simulink model "controller_template_ObsAvoid"  (Simulink 7.8)
settings: Solver=FixedStepDiscrete  SolverMode=SingleTasking  StartTime=0.0  StopTime=inf  FixedStep=Ts  RelTol=1e-3
PreLoadFcn:
  | load_waypoints
  | main;
StopFcn:
  | y_ref_wall = RecordYZ.signals(1).values(:,2);
  | y_wall = RecordYZ.signals(1).values(:,1);
  | 
  | z_ref_wall = RecordYZ.signals(2).values(:,2);
  | z_wall = RecordYZ.signals(2).values(:,1);
  | 
  | close all;
  | figure;
  | plot(y_ref_wall,z_ref_wall,'b','LineWidth',2); hold on;
  | plot(y_wall,z_wall,'r','LineWidth',2); grid on;
  | plot(traj_FG.X_ref_y_real(1,:),-traj_FG.X_ref_z_real(1,:),'o-g');
  | axis equal;
values from neighbouring files (symbols this model uses):
  Fi_Yaw = [-1.14619813144 0 0]    [kostas_malakies.mat]    (also in kostas_malakies2.mat; matlab.mat = -0.284754025426)
  Fi_Zdir = [0 -1.80359099426e-16 0 1.4149586889 0 0 2.30859647265e-14 -5.77149118162e-15 0 0 0 0 ... (54 elements, 27x2)]    [kostas_malakies.mat]    (also in kostas_malakies2.mat = [4.30976351396 0 4.73307471514 3.80948040666 0 0 0 0.5468933; matlab.mat = [0 -9.51943523339e-14 0 1.99761158231 0 1.18992940417e-14 0 )
  g = 9.8065    [kostas_malakies.mat]    (also in kostas_malakies2.mat; load_PMModel.m = 9.81; main.m; main_last.m)
  Gi_Yaw = [4.4408920985e-16 -3.14159265359 3.14159265359]    [kostas_malakies.mat]    (also in kostas_malakies2.mat = [-4.4408920985e-16 -3.14159265359 3.14159265359]; matlab.mat = 4.4408920985e-16)
  Gi_Zdir = [-1 -1 -1 2.22044604925e-16 -1 -1 -1 -1 1 -1 -1 -1 ... (27 elements, 27x1)]    [kostas_malakies.mat]    (also in kostas_malakies2.mat = [0.174387892495 -1 0.368373831608 3.33066907388e-16 -1 -1 -1; matlab.mat = [-2 -2 -2 1.11022302463e-15 -2 -2 -2 2 -2 -2 -2 2 ... (21 el)
  Hn_Yaw = [1 -1 -1 1 1 -1]    [kostas_malakies.mat]    (also in kostas_malakies2.mat; matlab.mat = [1 -1])
  Hn_Zdir = [-0.560552458797 -0.996815278536 -0.988320507921 0.666673243042 -1 0 -0.421994354267 -0.987440631917 -0.973284290019 -0.956170964903 -0.936236606521 0.560552458797 ... (224 elements, 112x2)]    [kostas_malakies.mat]    (also in kostas_malakies2.mat = [-0.781813705838 -0.712499731132 0.751798766698 0 -0.7286973; matlab.mat = [1 -1 -0.996815278536 -0.990718937584 -0.276007160242 0.3840)
  kalm_mpc_yaw =     [kostas_malakies.mat]    (also in kostas_malakies2.mat)
  Kn_Yaw = [2.74088097634 2.74088097634 -2.74088097634 3.14159265359 -2.74088097634 3.14159265359]    [kostas_malakies.mat]    (also in kostas_malakies2.mat; matlab.mat = [0.0873 0.0873])
  Kn_Zdir = [0.727672356179 1.00172267683 1.00656919451 -0.471160923828 1 1 1.18526984431 1.00688561667 1.01272393898 1.01603878926 1.01572683497 -0.727672356179 ... (112 elements, 112x1)]    [kostas_malakies.mat]    (also in kostas_malakies2.mat = [0.21304012328 0.326509029469 -0.262060822346 1 0.301409884 ; matlab.mat = [1 1 1.00663007512 1.02122194908 0.632590992205 -0.384463644)
  MAX_BIAS_YAW_RATE = 0.0872664625997    [kostas_malakies.mat]    (also in kostas_malakies2.mat; main.m; main_last.m)
  Nc_Yaw = [2 2 2]    [kostas_malakies.mat]    (also in kostas_malakies2.mat; matlab.mat = 2)
  Nc_Zdir = [6 7 3 6 3 4 4 3 6 5 3 4 ... (27 elements, 27x1)]    [kostas_malakies.mat]    (also in kostas_malakies2.mat = [4 4 3 12 5 4 3 3 4 3 3 4 ... (93 elements, 93x1)]; matlab.mat = [6 3 7 4 4 3 4 6 3 5 3 3 ... (21 elements, 21x1)])
  pitch_cmd2pitch_1stOrd = 1.42468924998    [kostas_malakies.mat]    (also in kostas_malakies2.mat)
  roll_cmd2roll_1stOrd = 1.38101661575    [kostas_malakies.mat]    (also in kostas_malakies2.mat)
  thrust_cmd2thrust_0thOrd = 0.876575459522    [kostas_malakies.mat]    (also in kostas_malakies2.mat)
  THRUST_CMD_GAIN = -0.0835    [kostas_malakies.mat]    (also in kostas_malakies2.mat; load_PMModel.m)
  traj_FG =     [kostas.mat]    (also in kostas_malakies.mat; kostas_malakies2.mat; main.m = ReferenceCreator(maxdisty,maxdistz,scale_y,scale_z); main_last.m = ReferenceCreator(maxdisty,maxdistz,scale_y,scale_z))
  Ts = 0.02    [kostas_malakies.mat]    (also in kostas_malakies2.mat; main.m; main_last.m; matlab.mat = 0.08)
  yaw_cmd2yaw_1stOrd = 2.01792090263    [kostas_malakies.mat]    (also in kostas_malakies2.mat)
  z = [-0.93079906702 -0.933865725994 -0.937557637691 -0.939011216164 -0.94143640995 -0.944628417492 -0.947235524654 -0.949601888657 -0.952827751637 -0.9567258358 -0.958320975304 -0.960991024971 ... (7988 elements, 7988x1)]    [kostas_malakies2.mat]    (also in plotDataTest.m = simout_data.signals.values(:,11))
undefined symbols (not defined in the file or in its folder): XYctrl
libraries: simulink x44, Hquad_control_LIB_MPC x13
(part 2 of 2)

== system controller_template_ObsAvoid/FreeFlight Pos Ctrl/MAIN CONTROL LOOP1/z controller MPC FG ==
  reset : Inport  PortDimensions=1
  X_ref_z : Inport  Port=2
  "z_states_est  " : Inport  Port=3
  Add : Sum  Inputs=+-
  Demux : Demux  Outputs=3
  Display : Display
  Display1 : Display
  Explicit Ctrl1 : Subsystem
  Mean : Subsystem
  Mux : Mux  Inputs=3
  Saturation : Saturate  UpperLimit=1  LowerLimit=-1
  Saturation1 : Saturate  UpperLimit=1  LowerLimit=-1
  Saturation2 : Saturate  UpperLimit=1  LowerLimit=-1
  Slider Gain : simulink/Math Operations/Slider Gain  low=0  gain=1.1  high=2
  Subsystem : Subsystem
  Wall Deviation : Subsystem
  thrust_cmd : Outport  PortDimensions=1
  wires:
  "z_states_est  "/1 -> Demux/1
  Demux/2 -> Saturation/1
  Demux/1 -> Add/1
  X_ref_z/1 -> Add/2
  Add/1 -> Saturation1/1
  Mux/1 -> Explicit Ctrl1/1(States)
  Saturation/1 -> Mux/2
  Saturation1/1 -> Display/1, Mux/1, Subsystem/3(dz)
  Mean/1(u_mean) -> thrust_cmd/1, Display1/1
  Saturation2/1 -> Mean/1(u)
  Demux/3 -> Wall Deviation/1(posx)
  Wall Deviation/1(deltax) -> Mux/3, Subsystem/2(dx)
  Explicit Ctrl1/1(Input) -> Subsystem/1(u_thrust)
  Subsystem/1(u_thrust_out) -> Slider Gain/1
  Slider Gain/1 -> Saturation2/1

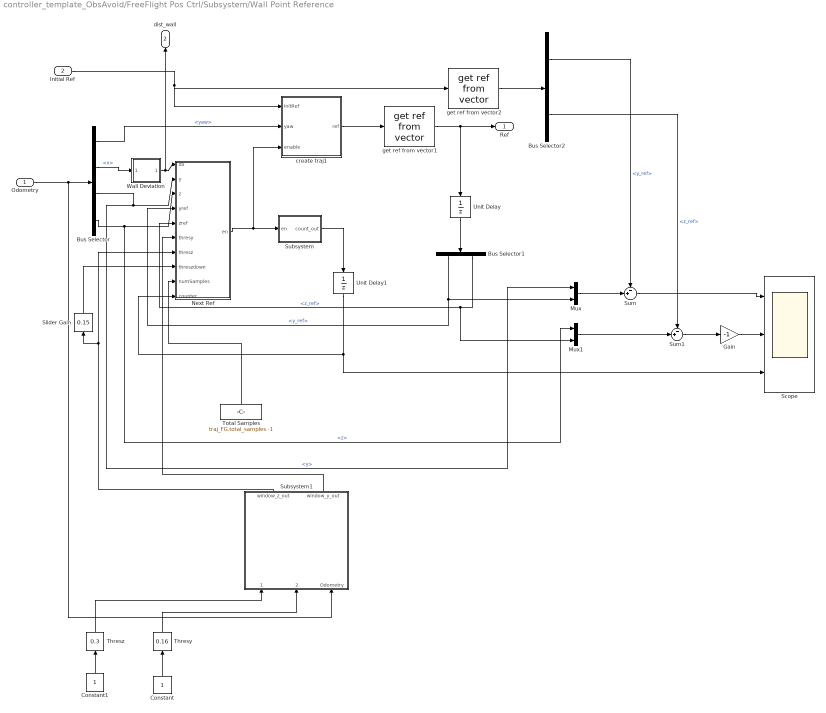
== system controller_template_ObsAvoid/FreeFlight Pos Ctrl/Subsystem/Wall Point Reference ==
  Odometry : Inport
  Initial Ref : Inport  Port=2
  Bus Selector : BusSelector  OutputSignals=rpy.yaw,pos.x,pos.y,pos.z
  Bus Selector1 : BusSelector  OutputSignals=pose_ref.y_ref,pose_ref.z_ref
  Bus Selector2 : BusSelector  OutputSignals=pose_ref.y_ref,pose_ref.z_ref
  Constant : Constant
  Constant1 : Constant
  Gain : Gain  Gain=-1
  Mux : Mux  Inputs=2
  Mux1 : Mux  Inputs=2
  Next Ref : MATLAB Function  TreatAsAtomicUnit=on
  Scope : Scope  NumInputPorts=3
      settings: YMin=0.575~-0.125~58  YMax=1.125~0.275~64  SaveName=RecordYZ
  Slider Gain : simulink/Math Operations/Slider Gain  low=0  gain=0.15  high=2
  Subsystem : Subsystem
  Subsystem1 : Subsystem
  Sum : Sum  Inputs=-+|
  Sum1 : Sum  Inputs=-+|
  Thresy : simulink/Math Operations/Slider Gain  low=0  gain=0.16  high=1
  Thresz : simulink/Math Operations/Slider Gain  low=0  gain=0.3  high=2
  Total Samples : Constant  Value=traj_FG.total_samples -1
  Unit Delay : UnitDelay  SampleTime=-1
  Unit Delay1 : UnitDelay  SampleTime=-1
  Wall Deviation : Subsystem
  create traj1 : Subsystem
  get ref from vector1 : Hquad_control_LIB_MPC/pos controller/get ref from vector
  get ref from vector2 : Hquad_control_LIB_MPC/pos controller/get ref from vector
  Ref : Outport
  dist_wall : Outport  Port=2
  wires:
  get ref from vector1/1 -> Ref/1, Unit Delay/1
  create traj1/1(ref) -> get ref from vector1/1
  Initial Ref/1 -> create traj1/1(InitRef), get ref from vector2/1
  Odometry/1 -> Bus Selector/1, Subsystem1/3(Odometry)
  Bus Selector/1 -> create traj1/2(yaw)  "<yaw>"
  Bus Selector/3 -> Next Ref/2(y), Mux/1  "<y>"
  Bus Selector/4 -> Next Ref/3(z), Mux1/1  "<z>"
  Unit Delay/1 -> Bus Selector1/1
  Bus Selector1/1 -> Next Ref/4(yref), Mux/2  "<y_ref>"
  Bus Selector1/2 -> Next Ref/5(zref), Mux1/2  "<z_ref>"
  Constant/1 -> Thresy/1
  Thresy/1 -> Subsystem1/2(nominal_window_y)
  Next Ref/1(en) -> create traj1/3(enable), Subsystem/1(en)
  Wall Deviation/1(deltax) -> Next Ref/1(dx), dist_wall/1
  Bus Selector/2 -> Wall Deviation/1(posx)  "<x>"
  Total Samples/1 -> Next Ref/9(numSamples)
  Unit Delay1/1 -> Next Ref/10(counter), Scope/3
  Subsystem/1(count_out) -> Unit Delay1/1
  Constant1/1 -> Thresz/1
  Thresz/1 -> Subsystem1/1(nominal_window_z)
  Gain/1 -> Scope/2
  Mux/1 -> Sum/2
  Mux1/1 -> Sum1/2
  Sum1/1 -> Gain/1
  Sum/1 -> Scope/1
  get ref from vector2/1 -> Bus Selector2/1
  Bus Selector2/1 -> Sum/1  "<y_ref>"
  Bus Selector2/2 -> Sum1/1  "<z_ref>"
  Subsystem1/2(window_y_out) -> Next Ref/6(thresy)
  Subsystem1/1(window_z_out) -> Next Ref/7(thresz), Slider Gain/1
  Slider Gain/1 -> Next Ref/8(threszdown)

== system controller_template_ObsAvoid/FreeFlight Pos Ctrl/decoupling and rotation/decoupling  ==
  "roll_meas  " : Inport  PortDimensions=1
  "pitch_meas  " : Inport  Port=2  PortDimensions=1
  cmd : Inport  Port=3
  mass : Inport  Port=4
  posx : Inport  Port=5
  Bus Creator : BusCreator
  Bus Selector3 : BusSelector  OutputSignals=pitch_cmd,roll_cmd,thrust_cmd,yaw_rate_cmd
  Embedded MATLAB Function : MATLAB Function  TreatAsAtomicUnit=on
  Wall Deviation : Subsystem
  g : Constant  Value=g
  "cmd_comp  " : Outport
  wires:
  "roll_meas  "/1 -> Embedded MATLAB Function/2(roll_meas)
  "pitch_meas  "/1 -> Embedded MATLAB Function/1(pitch_meas)
  cmd/1 -> Bus Selector3/1
  Bus Selector3/4 -> Bus Creator/4  "<yaw_rate_cmd>"
  Bus Creator/1 -> "cmd_comp  "/1
  Embedded MATLAB Function/3(thrust_comp) -> Bus Creator/3  "thrust_cmd"
  Embedded MATLAB Function/2(roll_cmd_comp) -> Bus Creator/2  "roll_cmd"
  Embedded MATLAB Function/1(pitch_cmd_comp) -> Bus Creator/1  "pitch_cmd"
  Bus Selector3/1 -> Embedded MATLAB Function/3(pitch_cmd)  "<pitch_cmd>"
  Bus Selector3/2 -> Embedded MATLAB Function/4(roll_cmd)  "<roll_cmd>"
  Bus Selector3/3 -> Embedded MATLAB Function/5(thrust)  "<thrust_cmd>"
  mass/1 -> Embedded MATLAB Function/6(m)
  g/1 -> Embedded MATLAB Function/7(g)
  posx/1 -> Wall Deviation/1(posx)
  Wall Deviation/1(deltax) -> Embedded MATLAB Function/8(posx)

== system controller_template_ObsAvoid/FreeFlight Pos Ctrl/decoupling and rotation/rotate_to_quat_frame ==
  yaw_meas : Inport
  cmd_comp : Inport  Port=2
  bias : Inport  Port=3
  Bus Creator1 : BusCreator
  Bus Creator2 : BusCreator
  Bus Selector1 : BusSelector  OutputSignals=thrust_bias,yaw_rate_bias
  Bus Selector2 : BusSelector  OutputSignals=pitch_bias,roll_bias
  Bus Selector3 : BusSelector  OutputSignals=pitch_cmd,roll_cmd
  Bus Selector4 : BusSelector  OutputSignals=thrust_cmd,yaw_rate_cmd
  Embedded MATLAB Function : MATLAB Function  TreatAsAtomicUnit=on
  "cmd_rot  " : Outport
  bias_rot : Outport  Port=2
  wires:
  yaw_meas/1 -> Embedded MATLAB Function/1(yaw)
  bias/1 -> Bus Selector2/1, Bus Selector1/1
  Bus Creator1/1 -> bias_rot/1
  Bus Selector2/1 -> Embedded MATLAB Function/4(pitch_bias)  "<pitch_bias>"
  Bus Selector2/2 -> Embedded MATLAB Function/5(roll_bias)  "<roll_bias>"
  Embedded MATLAB Function/3(pitch_bias_rot) -> Bus Creator1/1  "pitch_bias"
  Embedded MATLAB Function/4(roll_bias_rot) -> Bus Creator1/2  "roll_bias"
  Bus Creator2/1 -> "cmd_rot  "/1
  Bus Selector3/2 -> Embedded MATLAB Function/3(roll_cmd)  "<roll_cmd>"
  Bus Selector3/1 -> Embedded MATLAB Function/2(pitch_cmd)  "<pitch_cmd>"
  cmd_comp/1 -> Bus Selector3/1, Bus Selector4/1
  Embedded MATLAB Function/1(pitch_rot) -> Bus Creator2/1  "pitch_cmd"
  Embedded MATLAB Function/2(roll_rot) -> Bus Creator2/2  "roll_cmd"
  Bus Selector4/1 -> Bus Creator2/3  "<thrust_cmd>"
  Bus Selector4/2 -> Bus Creator2/4  "<yaw_rate_cmd>"
  Bus Selector1/1 -> Bus Creator1/3  "<thrust_bias>"
  Bus Selector1/2 -> Bus Creator1/4  "<yaw_rate_bias>"

== system controller_template_ObsAvoid/pos controller/MAIN CONTROL LOOP1/demux ==
  odometry : Inport
  ref : Inport  Port=2
  reset : Inport  Port=3
  Bus Creator : BusCreator  Inputs=3
  Bus Creator1 : BusCreator  Inputs=3
  Bus Creator2 : BusCreator  Inputs=2
  Bus Creator3 : BusCreator  Inputs=2
  Bus Selector1 : BusSelector  OutputSignals=X_ref_x,X_ref_y,X_ref_z,X_ref_yaw
  Bus Selector2 : BusSelector  OutputSignals=pos.x,vel.x_dot,rpy.pitch,pos.y,vel.y_dot,rpy.roll,pos.z,vel.z_dot,rpy.yaw,ang_vel.ang_vel_z
  reset1 : Outport
  X_ref_x : Outport  Port=2
  x_states_meas : Outport  Port=3  PortDimensions=3
  reset2 : Outport  Port=4
  X_ref_y : Outport  Port=5
  y_states_meas : Outport  Port=6  PortDimensions=3
  reset3 : Outport  Port=7
  X_ref_z : Outport  Port=8
  z_states_meas : Outport  Port=9  PortDimensions=2
  reset4 : Outport  Port=10
  X_ref_yaw : Outport  Port=11
  yaw_states_meas : Outport  Port=12  PortDimensions=2
  wires:
  Bus Selector1/4 -> X_ref_yaw/1  "<X_ref_yaw>"
  Bus Selector1/3 -> X_ref_z/1  "<X_ref_z>"
  Bus Selector2/6 -> Bus Creator1/3  "<roll>"
  Bus Selector2/3 -> Bus Creator/3  "<pitch>"
  odometry/1 -> Bus Selector2/1
  Bus Creator/1 -> x_states_meas/1
  Bus Selector2/1 -> Bus Creator/1  "<x>"
  Bus Selector2/2 -> Bus Creator/2  "<x_dot>"
  Bus Selector2/4 -> Bus Creator1/1  "<y>"
  Bus Selector2/5 -> Bus Creator1/2  "<y_dot>"
  Bus Creator1/1 -> y_states_meas/1
  Bus Selector2/7 -> Bus Creator2/1  "<z>"
  Bus Selector2/8 -> Bus Creator2/2  "<z_dot>"
  Bus Selector2/9 -> Bus Creator3/1  "<yaw>"
  Bus Selector2/10 -> Bus Creator3/2  "<ang_vel_z>"
  Bus Creator2/1 -> z_states_meas/1
  Bus Creator3/1 -> yaw_states_meas/1
  ref/1 -> Bus Selector1/1
  Bus Selector1/1 -> X_ref_x/1  "<X_ref_x>"
  Bus Selector1/2 -> X_ref_y/1  "<X_ref_y>"
  reset/1 -> reset3/1, reset4/1, reset2/1, reset1/1

== system controller_template_ObsAvoid/pos controller/MAIN CONTROL LOOP1/yaw states estimator bias ==
  yaw_rate_cmd : Inport  PortDimensions=1
  yaw_states_meas : Inport  Port=2  PortDimensions=2
  yaw_rate_bias_in : Inport  Port=3  PortDimensions=1
  A : Constant  Value=kalm_mpc_yaw.A
  B : Constant  Value=kalm_mpc_yaw.B
  Bus Selector3 : BusSelector  OutputSignals=yaw,ang_vel_z
  C : Constant  Value=kalm_mpc_yaw.C
  D : Constant  Value=kalm_mpc_yaw.D
  Demux3 : Demux  Outputs=2
  Mux1 : Mux  Inputs=2
  Mux4 : Mux  Inputs=2
  Q : Constant  Value=kalm_mpc_yaw.Q
  R : Constant  Value=kalm_mpc_yaw.R
  Saturation : Saturate  UpperLimit=MAX_BIAS_YAW_RATE  LowerLimit=-MAX_BIAS_YAW_RATE
  Unit Delay External IC1 : simulink/Additional Math & Discrete/Additional Discrete/Unit Delay External IC  tsamp=-1
  Unit Delay1 : UnitDelay  X0=kalm_mpc_yaw.P  SampleTime=Ts
  discrete kalman filter : MATLAB Function  AncestorBlock=Hquad_control_LIB_LQRI/x states estimator/discrete kalman filter  TreatAsAtomicUnit=on
  yaw_states_est : Outport  PortDimensions=2
  yaw_rate_bias : Outport  Port=2  PortDimensions=1
  wires:
  Unit Delay External IC1/1 -> Mux1/1
  yaw_rate_bias_in/1 -> Mux1/2
  Mux1/1 -> discrete kalman filter/10(state)
  Saturation/1 -> yaw_rate_bias/1
  Demux3/1 -> yaw_states_est/1, Unit Delay External IC1/1
  Demux3/2 -> Saturation/1
  R/1 -> discrete kalman filter/6(R)
  Q/1 -> discrete kalman filter/5(Q)
  Mux4/1 -> discrete kalman filter/8(y), Unit Delay External IC1/2
  yaw_rate_cmd/1 -> discrete kalman filter/7(u)
  Unit Delay1/1 -> discrete kalman filter/9(P)
  discrete kalman filter/2(P_est) -> Unit Delay1/1
  discrete kalman filter/1(state_est) -> Demux3/1
  D/1 -> discrete kalman filter/4(D)
  C/1 -> discrete kalman filter/3(C)
  B/1 -> discrete kalman filter/2(B)
  A/1 -> discrete kalman filter/1(A)
  yaw_states_meas/1 -> Bus Selector3/1
  Bus Selector3/1 -> Mux4/1  "<yaw>"
  Bus Selector3/2 -> Mux4/2  "<ang_vel_z>"

== system controller_template_ObsAvoid/FreeFlight Pos Ctrl/MAIN CONTROL LOOP1/x controller MPC FG  1/Explicit Ctrl Free Flight1 ==
  States : Inport
  Rate Transition : RateTransition  OutPortSampleTime=0.08
  Subsystem : Subsystem
  pitch_cmd : Outport
  roll_cmd : Outport  Port=2
  flag_oob : Outport  Port=3
  wires:
  Subsystem/1(U_x) -> pitch_cmd/1
  States/1 -> Rate Transition/1
  Rate Transition/1 -> Subsystem/1(xy_state)
  Subsystem/2(U_y) -> roll_cmd/1
  Subsystem/3(flag_oob) -> flag_oob/1

== system controller_template_ObsAvoid/FreeFlight Pos Ctrl/MAIN CONTROL LOOP1/x controller MPC FG  1/Free Flight ==
  posx : Inport
  refx : Inport  Port=2
  Add : Sum  Inputs=+-
  Saturation3 : Saturate  UpperLimit=1  LowerLimit=-1
  deltax : Outport
  wires:
  refx/1 -> Add/2
  Saturation3/1 -> deltax/1
  Add/1 -> Saturation3/1
  posx/1 -> Add/1

== system controller_template_ObsAvoid/FreeFlight Pos Ctrl/MAIN CONTROL LOOP1/x controller MPC FG  1/Mean ==
  u : Inport
  Gain : Gain  Gain=.33333
  Sum : Sum  Inputs=|++
  Sum1 : Sum  Inputs=|++
  Unit Delay : UnitDelay  SampleTime=-1
  Unit Delay1 : UnitDelay  SampleTime=-1
  Unit Delay2 : UnitDelay  SampleTime=-1
  u_mean : Outport
  wires:
  Unit Delay2/1 -> Sum1/1
  Sum1/1 -> Sum/2
  Unit Delay/1 -> Sum1/2
  Unit Delay1/1 -> Unit Delay/1
  Gain/1 -> Unit Delay2/1, Unit Delay1/1, u_mean/1
  Sum/1 -> Gain/1
  u/1 -> Sum/1

== system controller_template_ObsAvoid/FreeFlight Pos Ctrl/MAIN CONTROL LOOP1/x controller MPC FG  1/Mean1 ==
  u : Inport
  Gain : Gain  Gain=.33333
  Sum : Sum  Inputs=|++
  Sum1 : Sum  Inputs=|++
  Unit Delay : UnitDelay  SampleTime=-1
  Unit Delay1 : UnitDelay  SampleTime=-1
  Unit Delay2 : UnitDelay  SampleTime=-1
  u_mean : Outport
  wires:
  u/1 -> Sum/1
  Sum/1 -> Gain/1
  Gain/1 -> u_mean/1, Unit Delay1/1, Unit Delay2/1
  Unit Delay1/1 -> Unit Delay/1
  Unit Delay/1 -> Sum1/2
  Sum1/1 -> Sum/2
  Unit Delay2/1 -> Sum1/1

== system controller_template_ObsAvoid/FreeFlight Pos Ctrl/MAIN CONTROL LOOP1/x controller MPC FG  1/Wall Deviation ==
  posx : Inport
  Add : Sum  Inputs=+-
  Constant : Constant
  Constant1 : Constant
  MATLAB Function : MATLAB Function  TreatAsAtomicUnit=on
  Saturation3 : Saturate  UpperLimit=0  LowerLimit=-3
  Slider Gain : simulink/Math Operations/Slider Gain  low=-0.4  gain=2.56  high=3
  Slider Gain2 : simulink/Math Operations/Slider Gain  low=-0.4  gain=-0.05  high=2.95
  deltax : Outport
  wires:
  Slider Gain/1 -> Add/2
  Constant/1 -> Slider Gain/1
  Saturation3/1 -> deltax/1
  MATLAB Function/1(y) -> Saturation3/1
  Add/1 -> MATLAB Function/1(u)
  Slider Gain2/1 -> MATLAB Function/2(thres)
  Constant1/1 -> Slider Gain2/1
  posx/1 -> Add/1

== system controller_template_ObsAvoid/FreeFlight Pos Ctrl/MAIN CONTROL LOOP1/yaw controller MPC FG/Explicit Ctrl1 ==
  States : Inport
  input : Inport  Port=2
  Constant : Constant  Value=Hn_Yaw
  Constant1 : Constant  Value=Kn_Yaw
  Constant2 : Constant  Value=Fi_Yaw
  Constant3 : Constant  Value=Gi_Yaw
  Constant4 : Constant  Value=Nc_Yaw
  Ctrl_Xdir : MATLAB Function  TreatAsAtomicUnit=on
  Display : Display
  Rate Transition : RateTransition  OutPortSampleTime=0.02
  Rate Transition1 : RateTransition  OutPortSampleTime=0.02
  Unit Delay2 : UnitDelay  SampleTime=-1
  YawPropagate : Subsystem
  Input : Outport
  flag_oob : Outport  Port=2
  wires:
  Ctrl_Xdir/2(flag_oob) -> flag_oob/1
  Ctrl_Xdir/1(U) -> Input/1
  Constant4/1 -> Ctrl_Xdir/6(Nc)
  Constant3/1 -> Ctrl_Xdir/5(Gi)
  Constant2/1 -> Ctrl_Xdir/4(Fi)
  Constant1/1 -> Ctrl_Xdir/3(Kn)
  Constant/1 -> Ctrl_Xdir/2(Hn)
  States/1 -> Rate Transition/1
  Unit Delay2/1 -> YawPropagate/1(uprev)
  Rate Transition/1 -> YawPropagate/2(x)
  YawPropagate/1(Out1) -> Ctrl_Xdir/1(X), Display/1
  input/1 -> Rate Transition1/1
  Rate Transition1/1 -> Unit Delay2/1

== system controller_template_ObsAvoid/FreeFlight Pos Ctrl/MAIN CONTROL LOOP1/yaw controller MPC FG/Mean ==
  u : Inport
  Gain : Gain  Gain=.33333
  Sum : Sum  Inputs=|++
  Sum1 : Sum  Inputs=|++
  Unit Delay : UnitDelay  SampleTime=-1
  Unit Delay1 : UnitDelay  SampleTime=-1
  Unit Delay2 : UnitDelay  SampleTime=-1
  u_mean : Outport
  wires:
  u/1 -> Sum/1
  Sum/1 -> Gain/1
  Gain/1 -> u_mean/1, Unit Delay1/1, Unit Delay2/1
  Unit Delay1/1 -> Unit Delay/1
  Unit Delay/1 -> Sum1/2
  Sum1/1 -> Sum/2
  Unit Delay2/1 -> Sum1/1

== system controller_template_ObsAvoid/FreeFlight Pos Ctrl/MAIN CONTROL LOOP1/z controller MPC FG/Explicit Ctrl1 ==
  States : Inport
  Constant : Constant  Value=Hn_Zdir
  Constant1 : Constant  Value=Kn_Zdir
  Constant2 : Constant  Value=Fi_Zdir
  Constant3 : Constant  Value=Gi_Zdir
  Constant4 : Constant  Value=Nc_Zdir
  Ctrl_Xdir : MATLAB Function  TreatAsAtomicUnit=on
  Rate Transition : RateTransition  OutPortSampleTime=Tsz
  Input : Outport
  flag_oob : Outport  Port=2
  wires:
  Ctrl_Xdir/2(flag_oob) -> flag_oob/1
  Rate Transition/1 -> Ctrl_Xdir/1(X)
  Ctrl_Xdir/1(U) -> Input/1
  Constant4/1 -> Ctrl_Xdir/6(Nc)
  Constant3/1 -> Ctrl_Xdir/5(Gi)
  Constant2/1 -> Ctrl_Xdir/4(Fi)
  Constant1/1 -> Ctrl_Xdir/3(Kn)
  Constant/1 -> Ctrl_Xdir/2(Hn)
  States/1 -> Rate Transition/1

== system controller_template_ObsAvoid/FreeFlight Pos Ctrl/MAIN CONTROL LOOP1/z controller MPC FG/Mean ==
  u : Inport
  Gain : Gain  Gain=.33333
  Sum : Sum  Inputs=|++
  Sum1 : Sum  Inputs=|++
  Unit Delay : UnitDelay  SampleTime=-1
  Unit Delay1 : UnitDelay  SampleTime=-1
  Unit Delay2 : UnitDelay  SampleTime=-1
  u_mean : Outport
  wires:
  u/1 -> Sum/1
  Sum/1 -> Gain/1
  Gain/1 -> u_mean/1, Unit Delay1/1, Unit Delay2/1
  Unit Delay1/1 -> Unit Delay/1
  Unit Delay/1 -> Sum1/2
  Sum1/1 -> Sum/2
  Unit Delay2/1 -> Sum1/1

== system controller_template_ObsAvoid/FreeFlight Pos Ctrl/MAIN CONTROL LOOP1/z controller MPC FG/Subsystem ==
  u_thrust : Inport
  dx : Inport  Port=2
  dz : Inport  Port=3
  Constant : Constant
  MATLAB Function : MATLAB Function  TreatAsAtomicUnit=on
  Slider Gain : simulink/Math Operations/Slider Gain  low=0  gain=1  high=2
  u_thrust_out : Outport
  wires:
  u_thrust/1 -> MATLAB Function/1(u_thrust)
  dx/1 -> MATLAB Function/2(dx)
  dz/1 -> MATLAB Function/3(dz)
  Slider Gain/1 -> MATLAB Function/4(K_g_up)
  Constant/1 -> Slider Gain/1
  MATLAB Function/1(u_thrust_out) -> u_thrust_out/1

== system controller_template_ObsAvoid/FreeFlight Pos Ctrl/MAIN CONTROL LOOP1/z controller MPC FG/Wall Deviation ==
  posx : Inport
  Add : Sum  Inputs=+-
  Constant : Constant
  Constant1 : Constant
  MATLAB Function : MATLAB Function  TreatAsAtomicUnit=on
  Saturation3 : Saturate  UpperLimit=.1  LowerLimit=-1
  Slider Gain : simulink/Math Operations/Slider Gain  low=-0.4  gain=2.97  high=3
  Slider Gain2 : simulink/Math Operations/Slider Gain  low=-0.4  gain=-0.07  high=2.95
  deltax : Outport
  wires:
  posx/1 -> Add/1
  Constant1/1 -> Slider Gain2/1
  Slider Gain2/1 -> MATLAB Function/2(thres)
  Add/1 -> MATLAB Function/1(u)
  MATLAB Function/1(y) -> Saturation3/1
  Saturation3/1 -> deltax/1
  Constant/1 -> Slider Gain/1
  Slider Gain/1 -> Add/2

== system controller_template_ObsAvoid/FreeFlight Pos Ctrl/Subsystem/Wall Point Reference/Subsystem ==
  en : Inport
  MATLAB Function : MATLAB Function  TreatAsAtomicUnit=on
  Unit Delay : UnitDelay  SampleTime=-1
  Unit Delay1 : UnitDelay  SampleTime=-1
  count_out : Outport
  wires:
  en/1 -> MATLAB Function/1(en_flag), Unit Delay/1
  Unit Delay/1 -> MATLAB Function/2(en_flag_prev)
  MATLAB Function/1(count_out) -> Unit Delay1/1, count_out/1
  Unit Delay1/1 -> MATLAB Function/3(count_out_prev)

== system controller_template_ObsAvoid/FreeFlight Pos Ctrl/Subsystem/Wall Point Reference/Subsystem1 ==
  nominal_window_z : Inport
  nominal_window_y : Inport  Port=2
  Odometry : Inport  Port=3
  Bus Selector : BusSelector  OutputSignals=vel.z_dot,vel.y_dot
  Constant{,1..3} (4 alike) : Constant
  MATLAB Function : MATLAB Function  TreatAsAtomicUnit=on
  Scope : Scope  NumInputPorts=2
      settings: YMin=0.3~0.15  YMax=0.3~0.15  SaveName=ScopeData16
  Slider Gain : simulink/Math Operations/Slider Gain  low=0  gain=0.0515  high=2
  Slider Gain1 : simulink/Math Operations/Slider Gain  low=0  gain=10.065  high=10.065
  Slider Gain2 : simulink/Math Operations/Slider Gain  low=0  gain=1  high=2
  Slider Gain3 : simulink/Math Operations/Slider Gain  low=0  gain=0.095  high=2
  Slider Gain4 : simulink/Math Operations/Slider Gain  low=0  gain=0  high=2
  Switch : Switch  Threshold=0.5
  Switch1 : Switch  Threshold=0.5
  window_z_out : Outport
  window_y_out : Outport  Port=2
  wires:
  nominal_window_z/1 -> MATLAB Function/1(nominal_window_z), Switch/3
  nominal_window_y/1 -> MATLAB Function/2(nominal_window_y), Switch1/3
  Slider Gain/1 -> MATLAB Function/5(thres_vel_z)
  Constant/1 -> Slider Gain/1, Slider Gain1/1
  Slider Gain1/1 -> MATLAB Function/6(thres_vel_y)
  Slider Gain2/1 -> MATLAB Function/7(K_gain)
  Constant1/1 -> Slider Gain2/1
  Slider Gain3/1 -> MATLAB Function/8(maxDeltaWindow)
  Constant2/1 -> Slider Gain3/1
  MATLAB Function/1(nominal_window_z_out) -> Switch/1
  Switch/1 -> window_z_out/1, Scope/1
  MATLAB Function/2(nominal_window_y_out) -> Switch1/1
  Switch1/1 -> window_y_out/1, Scope/2
  Constant3/1 -> Slider Gain4/1
  Slider Gain4/1 -> Switch/2, Switch1/2
  Odometry/1 -> Bus Selector/1
  Bus Selector/1 -> MATLAB Function/3(vel_z)  "<z_dot>"
  Bus Selector/2 -> MATLAB Function/4(vel_y)  "<y_dot>"

== system controller_template_ObsAvoid/FreeFlight Pos Ctrl/Subsystem/Wall Point Reference/Wall Deviation ==
  posx : Inport
  Add : Sum  Inputs=+-
  Constant : Constant
  Constant1 : Constant
  MATLAB Function : MATLAB Function  TreatAsAtomicUnit=on
  Saturation3 : Saturate  UpperLimit=0  LowerLimit=-1
  Slider Gain : simulink/Math Operations/Slider Gain  low=-0.4  gain=2.97  high=3
  Slider Gain2 : simulink/Math Operations/Slider Gain  low=-0.4  gain=-0.07  high=2.95
  deltax : Outport
  wires:
  posx/1 -> Add/1
  Constant1/1 -> Slider Gain2/1
  Slider Gain2/1 -> MATLAB Function/2(thres)
  Add/1 -> MATLAB Function/1(u)
  MATLAB Function/1(y) -> Saturation3/1
  Saturation3/1 -> deltax/1
  Constant/1 -> Slider Gain/1
  Slider Gain/1 -> Add/2

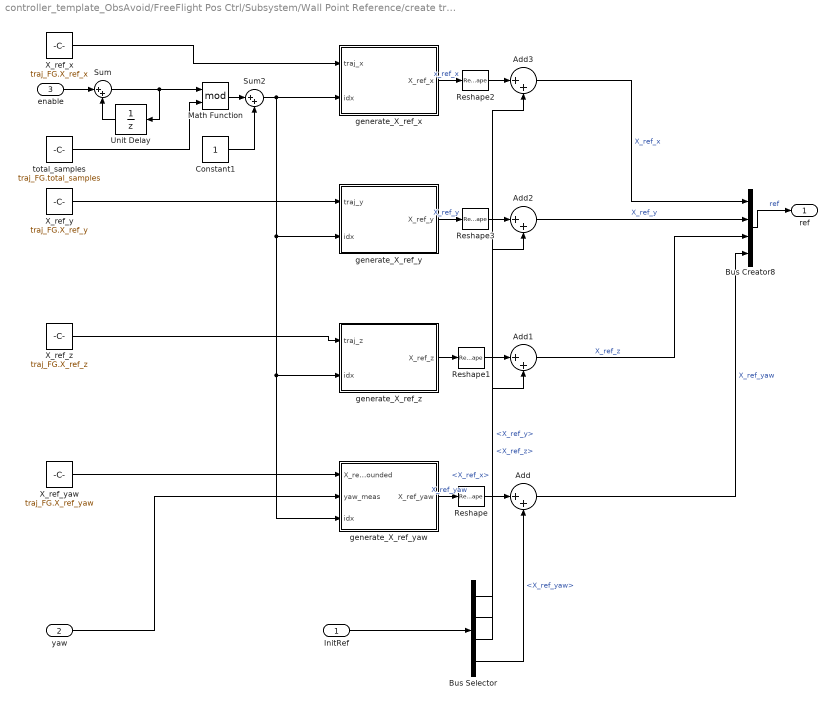
== system controller_template_ObsAvoid/FreeFlight Pos Ctrl/Subsystem/Wall Point Reference/create traj1 ==
  InitRef : Inport
  yaw : Inport  Port=2
  enable : Inport  Port=3
  Add{,1..3} (4 alike) : Sum  Inputs=|++
  Bus Creator8 : BusCreator
  Bus Selector : BusSelector  OutputSignals=X_ref_x,X_ref_y,X_ref_z,X_ref_yaw
  Constant1 : Constant
  Math Function : Math  Operator=mod  SaturateOnIntegerOverflow=on
  Reshape{,1..3} (4 alike) : Reshape
  Sum : Sum  Inputs=|++
  Sum2 : Sum  Inputs=|++
  Unit Delay : UnitDelay  SampleTime=-1
  X_ref_x : Constant  Value=traj_FG.X_ref_x
  X_ref_y : Constant  Value=traj_FG.X_ref_y
  X_ref_yaw : Constant  Value=traj_FG.X_ref_yaw
  X_ref_z : Constant  Value=traj_FG.X_ref_z
  generate_X_ref_x : MATLAB Function  TreatAsAtomicUnit=on
  generate_X_ref_y : MATLAB Function  TreatAsAtomicUnit=on
  generate_X_ref_yaw : MATLAB Function  TreatAsAtomicUnit=on
  generate_X_ref_z : MATLAB Function  TreatAsAtomicUnit=on
  total_samples : Constant  Value=traj_FG.total_samples
  ref : Outport
  wires:
  Bus Creator8/1 -> ref/1  "ref"
  enable/1 -> Sum/1
  Unit Delay/1 -> Sum/2
  Sum/1 -> Unit Delay/1, Math Function/1
  total_samples/1 -> Math Function/2
  Math Function/1 -> Sum2/1
  Constant1/1 -> Sum2/2
  yaw/1 -> generate_X_ref_yaw/2(yaw_meas)
  Sum2/1 -> generate_X_ref_x/2(idx), generate_X_ref_yaw/3(idx), generate_X_ref_z/2(idx), generate_X_ref_y/2(idx)
  X_ref_y/1 -> generate_X_ref_y/1(traj_y)
  X_ref_x/1 -> generate_X_ref_x/1(traj_x)
  X_ref_yaw/1 -> generate_X_ref_yaw/1(X_ref_yaw_unbounded)
  X_ref_z/1 -> generate_X_ref_z/1(traj_z)
  InitRef/1 -> Bus Selector/1
  generate_X_ref_yaw/1(X_ref_yaw) -> Reshape/1  "X_ref_yaw"
  Add/1 -> Bus Creator8/4  "X_ref_yaw"
  generate_X_ref_x/1(X_ref_x) -> Reshape2/1  "x_ref_x"
  Add3/1 -> Bus Creator8/1  "X_ref_x"
  generate_X_ref_y/1(X_ref_y) -> Reshape3/1  "X_ref_y"
  Add2/1 -> Bus Creator8/2  "X_ref_y"
  generate_X_ref_z/1(X_ref_z) -> Reshape1/1
  Add1/1 -> Bus Creator8/3  "X_ref_z"
  Bus Selector/4 -> Add/2  "<X_ref_yaw>"
  Bus Selector/3 -> Add1/2  "<X_ref_z>"
  Bus Selector/2 -> Add2/2  "<X_ref_y>"
  Bus Selector/1 -> Add3/2  "<X_ref_x>"
  Reshape2/1 -> Add3/1
  Reshape3/1 -> Add2/1
  Reshape1/1 -> Add1/1
  Reshape/1 -> Add/1

== system controller_template_ObsAvoid/FreeFlight Pos Ctrl/decoupling and rotation/decoupling /Wall Deviation ==
  posx : Inport
  Add : Sum  Inputs=+-
  Constant : Constant
  Constant1 : Constant
  MATLAB Function : MATLAB Function  TreatAsAtomicUnit=on
  Saturation3 : Saturate  UpperLimit=0  LowerLimit=-1
  Slider Gain : simulink/Math Operations/Slider Gain  low=-0.4  gain=2.97  high=3
  Slider Gain2 : simulink/Math Operations/Slider Gain  low=-0.4  gain=-0.05  high=2.95
  deltax : Outport
  wires:
  posx/1 -> Add/1
  Constant1/1 -> Slider Gain2/1
  Slider Gain2/1 -> MATLAB Function/2(thres)
  Add/1 -> MATLAB Function/1(u)
  MATLAB Function/1(y) -> Saturation3/1
  Saturation3/1 -> deltax/1
  Constant/1 -> Slider Gain/1
  Slider Gain/1 -> Add/2

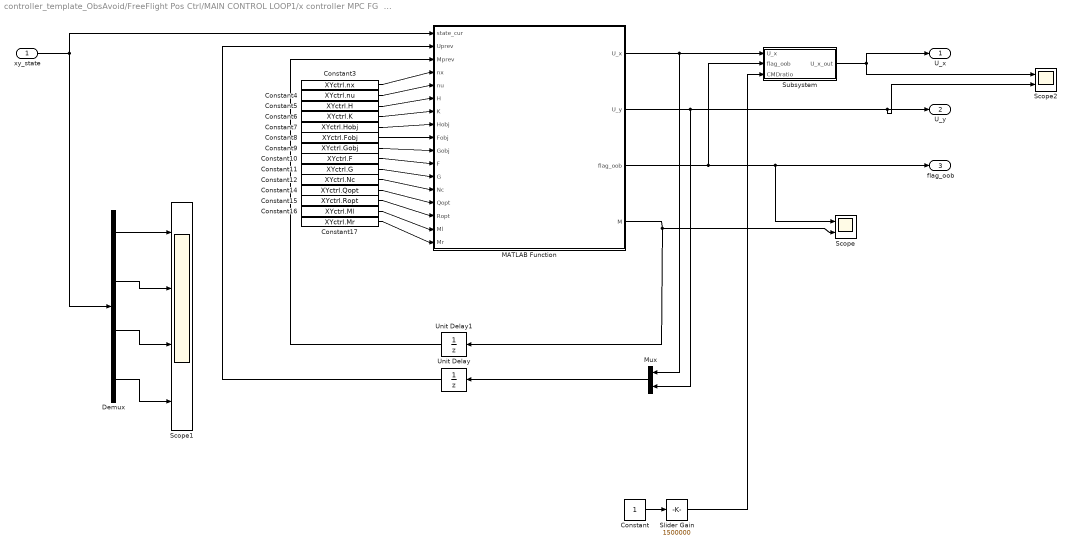
== system controller_template_ObsAvoid/FreeFlight Pos Ctrl/MAIN CONTROL LOOP1/x controller MPC FG  1/Explicit Ctrl Free Flight1/Subsystem ==
  xy_state : Inport
  Constant : Constant
  Constant10 : Constant  Value=XYctrl.F  VectorParams1D=off
  Constant11 : Constant  Value=XYctrl.G  VectorParams1D=off
  Constant12 : Constant  Value=XYctrl.Nc  VectorParams1D=off
  Constant14 : Constant  Value=XYctrl.Qopt  VectorParams1D=off
  Constant15 : Constant  Value=XYctrl.Ropt  VectorParams1D=off
  Constant16 : Constant  Value=XYctrl.Ml  VectorParams1D=off
  Constant17 : Constant  Value=XYctrl.Mr  VectorParams1D=off
  Constant3 : Constant  Value=XYctrl.nx  VectorParams1D=off
  Constant4 : Constant  Value=XYctrl.nu  VectorParams1D=off
  Constant5 : Constant  Value=XYctrl.H  VectorParams1D=off
  Constant6 : Constant  Value=XYctrl.K  VectorParams1D=off
  Constant7 : Constant  Value=XYctrl.Hobj  VectorParams1D=off
  Constant8 : Constant  Value=XYctrl.Fobj  VectorParams1D=off
  Constant9 : Constant  Value=XYctrl.Gobj  VectorParams1D=off
  Demux : Demux
  MATLAB Function : MATLAB Function  TreatAsAtomicUnit=on
  Mux : Mux  Inputs=2
  Scope : Scope  NumInputPorts=2
      settings: YMin=-5~1.9  YMax=5~2.1  SaveName=ScopeData20
  Scope1 : Scope  NumInputPorts=4
      settings: YMin=-2.2~-5~-1.2~-5  YMax=-1.925~5~-0.8~5  SaveName=ScopeData25
  Scope2 : Scope  NumInputPorts=2
      settings: YMin=-0.3~-5  YMax=0.35~5  SaveName=ScopeData26
  Slider Gain : simulink/Math Operations/Slider Gain  low=0  gain=1500000  high=1500000
  Subsystem : Subsystem
  Unit Delay : UnitDelay  SampleTime=-1
  Unit Delay1 : UnitDelay  X0=2  SampleTime=-1
  U_x : Outport
  U_y : Outport  Port=2
  flag_oob : Outport  Port=3
  wires:
  Constant3/1 -> MATLAB Function/4(nx)
  MATLAB Function/4(M) -> Unit Delay1/1, Scope/2
  Constant4/1 -> MATLAB Function/5(nu)
  Constant5/1 -> MATLAB Function/6(H)
  Constant6/1 -> MATLAB Function/7(K)
  Constant7/1 -> MATLAB Function/8(Hobj)
  Constant8/1 -> MATLAB Function/9(Fobj)
  Constant9/1 -> MATLAB Function/10(Gobj)
  Constant10/1 -> MATLAB Function/11(F)
  Constant11/1 -> MATLAB Function/12(G)
  Constant12/1 -> MATLAB Function/13(Nc)
  Constant14/1 -> MATLAB Function/14(Qopt)
  Constant15/1 -> MATLAB Function/15(Ropt)
  Constant16/1 -> MATLAB Function/16(Ml)
  Constant17/1 -> MATLAB Function/17(Mr)
  xy_state/1 -> MATLAB Function/1(state_cur), Demux/1
  Mux/1 -> Unit Delay/1
  MATLAB Function/1(U_x) -> Mux/1, Subsystem/1(U_x)
  MATLAB Function/2(U_y) -> Mux/2, U_y/1, Scope2/2
  Unit Delay/1 -> MATLAB Function/2(Uprev)
  Unit Delay1/1 -> MATLAB Function/3(Mprev)
  MATLAB Function/3(flag_oob) -> flag_oob/1, Scope/1, Subsystem/2(flag_oob)
  Demux/1 -> Scope1/1
  Demux/2 -> Scope1/2
  Demux/3 -> Scope1/3
  Demux/4 -> Scope1/4
  Subsystem/1(U_x_out) -> U_x/1, Scope2/1
  Constant/1 -> Slider Gain/1
  Slider Gain/1 -> Subsystem/3(CMDratio)

== system controller_template_ObsAvoid/FreeFlight Pos Ctrl/MAIN CONTROL LOOP1/yaw controller MPC FG/Explicit Ctrl1/YawPropagate ==
  uprev : Inport
  x : Inport  Port=2
  Constant : Constant
  Constant1 : Constant  Value=0
  MATLAB Function : MATLAB Function  TreatAsAtomicUnit=on
  Out1 : Outport
  wires:
  MATLAB Function/1(y) -> Out1/1
  x/1 -> MATLAB Function/1(x)
  uprev/1 -> MATLAB Function/4(u)
  Constant1/1 -> MATLAB Function/3(B)
  Constant/1 -> MATLAB Function/2(A)

== system controller_template_ObsAvoid/FreeFlight Pos Ctrl/MAIN CONTROL LOOP1/x controller MPC FG  1/Explicit Ctrl Free Flight1/Subsystem/Subsystem ==
  U_x : Inport
  flag_oob : Inport  Port=2
  CMDratio : Inport  Port=3
  MATLAB Function1 : MATLAB Function  TreatAsAtomicUnit=on
  Subsystem : Subsystem
  Subsystem1 : Subsystem
  U_x_out : Outport
  wires:
  U_x/1 -> Subsystem/1(In1)
  Subsystem/1(Out1) -> MATLAB Function1/1(U_x)
  Subsystem1/1(Out1) -> MATLAB Function1/2(flag_oob)
  CMDratio/1 -> MATLAB Function1/3(CMDratio)
  flag_oob/1 -> Subsystem1/1(In1)
  MATLAB Function1/1(U_x_out) -> U_x_out/1

== system controller_template_ObsAvoid/FreeFlight Pos Ctrl/MAIN CONTROL LOOP1/x controller MPC FG  1/Explicit Ctrl Free Flight1/Subsystem/Subsystem/Subsystem ==
  In1 : Inport
  Out1 : Outport  PortDimensions=1
  wires:
  In1/1 -> Out1/1

== system controller_template_ObsAvoid/FreeFlight Pos Ctrl/MAIN CONTROL LOOP1/x controller MPC FG  1/Explicit Ctrl Free Flight1/Subsystem/Subsystem/Subsystem1 ==
  In1 : Inport
  Out1 : Outport  PortDimensions=1
  wires:
  In1/1 -> Out1/1

== matlab function FreeFlight Pos Ctrl/MAIN CONTROL LOOP1/x controller MPC FG 1/Explicit Ctrl Free Flight1/Subsystem/Subsystem/MATLAB Function1 ==
  data: U_x input double; U_x_out output double; flag_oob input double; CMDratio input double
function U_x_out = fcn(U_x,flag_oob,CMDratio)
%#codegen

U_x_out = U_x;

if flag_oob == 1
    U_x_out = U_x/CMDratio;
end

end

== matlab function FreeFlight Pos Ctrl/MAIN CONTROL LOOP1/z controller MPC FG/Explicit Ctrl1/Ctrl_Xdir ==
  data: X input double; U output double; Hn input double; Kn input double; Fi input double; Gi input double; Nc input double; flag_oob output double
function [U,flag_oob] = OptimalMPCInput(X,Hn,Kn,Fi,Gi,Nc)

tolerance = 1;
nr  = size(Nc,1);
MPT_ABSTOL = 1e-8;
minreg = 0;
X = round(10000*X)/10000;

flag_oob = 0;
%maxSize = max(Nc);

Hi = zeros(100,3);
Ki = zeros(100,1);

% Find the proper region
abspos = 1;
for ireg = 1:nr
    sumViol = 0;
    isinside = 1;
    

  %  Hi(1:Nc(ireg),1:4) = Hn(abspos:(abspos+Nc(ireg)-1),1:4);
    for i = 1:Nc(ireg)
        for j = 1:3
            Hi(i,j) = Hn(abspos + i - 1,j);
        end
    end
    
%    Ki(1:Nc(ireg),1) = Kn(abspos:(abspos+Nc(ireg)-1),1);
    for i = 1:Nc(ireg)
        Ki(i,1) = Kn(abspos + i - 1,1);
    end
    abspos = abspos + Nc(ireg);
    
    F = Fi(ireg,:);
    G = Gi(ireg,:);
    
    nc = Nc(ireg);
    
    for ic = 1:nc
        hx = Hi(ic,:)*X;
        if ((hx - Ki(ic)) > MPT_ABSTOL)
            isinside = 0;
            sumViol = sumViol + (hx - Ki(ic));
        end
    end
    
    if (sumViol < tolerance)
        tolerance = sumViol;
        minreg = ireg;
    end
    % extract the right control law
    if (isinside == 1)
        U = F*X + G;
        return
    end
end
F = Fi(minreg,:);
G = Gi(minreg,:);
U = F*X + G;
flag_oob = 1;
%U = U_prev;
return

== matlab function FreeFlight Pos Ctrl/MAIN CONTROL LOOP1/yaw controller MPC FG/Explicit Ctrl1/Ctrl_Xdir ==
  data: X input double; U output double; Hn input double; Kn input double; Fi input double; Gi input double; Nc input double; flag_oob output double
function [U,flag_oob] = OptimalMPCInput(X,Hn,Kn,Fi,Gi,Nc)

tolerance = 1;
nr  = size(Nc,1);
MPT_ABSTOL = 1e-8;
minreg = 0;
X = round(10000*X)/10000;

flag_oob = 0;
%maxSize = max(Nc);

Hi = zeros(100,1);
Ki = zeros(100,1);

% Find the proper region
abspos = 1;
for ireg = 1:nr
    sumViol = 0;
    isinside = 1;
    

  %  Hi(1:Nc(ireg),1:4) = Hn(abspos:(abspos+Nc(ireg)-1),1:4);
    for i = 1:Nc(ireg)
        for j = 1:1
            Hi(i,j) = Hn(abspos + i - 1,j);
        end
    end
    
%    Ki(1:Nc(ireg),1) = Kn(abspos:(abspos+Nc(ireg)-1),1);
    for i = 1:Nc(ireg)
        Ki(i,1) = Kn(abspos + i - 1,1);
    end
    abspos = abspos + Nc(ireg);
    
    F = Fi(ireg,:);
    G = Gi(ireg,:);
    
    nc = Nc(ireg);
    
    for ic = 1:nc
        hx = Hi(ic,:)*X;
        if ((hx - Ki(ic)) > MPT_ABSTOL)
            isinside = 0;
            sumViol = sumViol + (hx - Ki(ic));
        end
    end
    
    if (sumViol < tolerance)
        tolerance = sumViol;
        minreg = ireg;
    end
    % extract the right control law
    if (isinside == 1)
        U = F*X + G;
        return
    end
end
F = Fi(minreg,:);
G = Gi(minreg,:);
U = F*X + G;
flag_oob = 1;
%U = U_prev;
return

== matlab function FreeFlight Pos Ctrl/MAIN CONTROL LOOP1/yaw controller MPC FG/Explicit Ctrl1/YawPropagate/MATLAB Function ==
  data: x input double; y output double; A input double; B input double; u input double
function y = fcn(x,A,B,u)
%#codegen

y = A*x + B*u;

== matlab function FreeFlight Pos Ctrl/Subsystem/Wall Point Reference/Wall Deviation/MATLAB Function ==
  data: u input double; y output double; thres input double
function y = fcn(u,thres)
%#codegen
if u >=thres
    y = 0;
else
    y = u;
end

== matlab function FreeFlight Pos Ctrl/decoupling and rotation/decoupling /Embedded MATLAB Function ==
  data: pitch_cmd_comp output double; roll_cmd_comp output double; pitch_meas input double; thrust_comp output double; roll_meas input double; pitch_cmd input double; roll_cmd input double; thrust input double; m input double; g input double; posx input double
function [pitch_cmd_comp, roll_cmd_comp, thrust_comp]  = fcn(pitch_meas, roll_meas, pitch_cmd, roll_cmd, thrust,m,g,posx)
%#eml
maxangle = 4*pi/180;
thrust_comp=thrust;
if (posx == 0)
    thrust_comp=thrust/(cos(pitch_meas)*cos(roll_meas));
    
    if abs(pitch_meas) >= maxangle && abs(roll_meas) >= maxangle
        thrust_comp=thrust/(cos(maxangle)*cos(maxangle));
    elseif abs(pitch_meas) >= maxangle
        thrust_comp=thrust/(cos(maxangle)*cos(roll_meas));
    elseif abs(roll_meas) >= maxangle
        thrust_comp=thrust/(cos(pitch_meas)*cos(maxangle));
    end
else
    thrust_comp=thrust/(cos(pitch_meas)*cos(roll_meas));
end
pitch_cmd_comp = m*g/thrust_comp*pitch_cmd;
roll_cmd_comp = m*g/thrust_comp*roll_cmd;

% pitch_cmd_comp=pitch_cmd;
% roll_cmd_comp=roll_cmd;
% pitch_cmd_comp = atan(Fx/(-thrust_comp));
% roll_cmd_comp = atan(Fy/(thrust_comp));

% pitch_cmd_comp = atan(-g*m*pitch_cmd/(-thrust));
% roll_cmd_comp = atan(g*m*roll_cmd*cos(pitch_meas)/(thrust));

== matlab function FreeFlight Pos Ctrl/decoupling and rotation/rotate_to_quat_frame/Embedded MATLAB Function ==
  data: yaw input double; pitch_rot output double; pitch_cmd input double; roll_cmd input double; pitch_bias input double; roll_bias input double; roll_rot output double; pitch_bias_rot output double; roll_bias_rot output double
function [pitch_rot,roll_rot, pitch_bias_rot,roll_bias_rot] = fcn(yaw, pitch_cmd, roll_cmd, pitch_bias, roll_bias)

sin_yaw=sin(yaw);
cos_yaw=cos(yaw);

R=[cos_yaw, sin_yaw; -sin_yaw, cos_yaw];

temp=R'*[pitch_cmd;roll_cmd];
pitch_rot=temp(1);
roll_rot=temp(2);

temp=R'*[pitch_bias;roll_bias];
pitch_bias_rot=temp(1);
roll_bias_rot=temp(2);

== matlab function FreeFlight Pos Ctrl/Subsystem/Wall Point Reference/Subsystem/MATLAB Function ==
  data: en_flag input double; count_out output double; en_flag_prev input double; count_out_prev input double
function count_out = fcn(en_flag,en_flag_prev,count_out_prev)
%#codegen

count_out = count_out_prev; 
if( ((en_flag == 1) && (en_flag_prev == 0)) || ((en_flag == 1) && (en_flag_prev == 1)) )
    count_out = count_out_prev + 1;
end

end

== matlab function FreeFlight Pos Ctrl/MAIN CONTROL LOOP1/Subsystem/MATLAB Function ==
  data: pitch_cmd input double; pitch_cmd_out output double; pitch_angle input double; dist_wall input double; K_gain input double; max_neg_pitch input double
function pitch_cmd_out = fcn(pitch_cmd,pitch_angle,dist_wall,K_gain,max_neg_pitch)
%#codegen

pitch_cmd_out = pitch_cmd;

if( (dist_wall == 0) && (pitch_angle < -max_neg_pitch) )
    pitch_cmd_out = pitch_cmd_out + K_gain*abs(pitch_angle + max_neg_pitch);
end

end

== matlab function FreeFlight Pos Ctrl/MAIN CONTROL LOOP1/z controller MPC FG/Wall Deviation/MATLAB Function ==
  data: u input double; y output double; thres input double
function y = fcn(u,thres)
%#codegen
if u >=thres
    y = 0.1;
else
    y = u;
end

== matlab function FreeFlight Pos Ctrl/MAIN CONTROL LOOP1/z controller MPC FG/Subsystem/MATLAB Function ==
  data: u_thrust input double; u_thrust_out output double; dx input double; dz input double; K_g_up input double
function u_thrust_out = fcn(u_thrust,dx,dz,K_g_up)
%#codegen

u_thrust_out = u_thrust;

if( dx>0 && dz<0 )
    u_thrust_out = K_g_up*u_thrust;
end

end

== matlab function FreeFlight Pos Ctrl/Subsystem/Wall Point Reference/Subsystem1/MATLAB Function ==
  data: nominal_window_z input double; nominal_window_z_out output double; nominal_window_y input double; vel_z input double; vel_y input double; thres_vel_z input double; thres_vel_y input double; K_gain input double; maxDeltaWindow input double; nominal_window_y_out output double
function [nominal_window_z_out,nominal_window_y_out] = fcn(nominal_window_z,nominal_window_y,vel_z,vel_y,thres_vel_z,thres_vel_y,K_gain,maxDeltaWindow)
%#codegen

nominal_window_z_out = nominal_window_z;
nominal_window_y_out = nominal_window_y;

vel_y = abs(vel_y);
vel_z = (vel_z);

if( vel_y > thres_vel_y )
    nominal_window_y_out = nominal_window_y - min(K_gain*abs(vel_y - thres_vel_y),maxDeltaWindow);
end

if( vel_z > thres_vel_z )
    nominal_window_z_out = nominal_window_z - min(K_gain*abs(vel_z - thres_vel_z),maxDeltaWindow);
end

end

== matlab function FreeFlight Pos Ctrl/Free Flight Reference/create traj/generate_X_ref_x ==
  data: traj_x input double; X_ref_x output double; idx input double
function X_ref_x  = fcn(traj_x,idx)

pred_horizon_x=30;

X_ref_x=traj_x(:,idx:idx+pred_horizon_x);

== matlab function FreeFlight Pos Ctrl/Free Flight Reference/create traj/generate_X_ref_y ==
  data: traj_y input double; X_ref_y output double; idx input double
function X_ref_y  = fcn(traj_y,idx)

pred_horizon_y=30;

X_ref_y=traj_y(:,idx:idx+pred_horizon_y);

== matlab function FreeFlight Pos Ctrl/Free Flight Reference/create traj/generate_X_ref_yaw ==
  data: X_ref_yaw_unbounded input double; X_ref_yaw output double; yaw_meas input double; idx input double
function X_ref_yaw  = fcn(X_ref_yaw_unbounded,yaw_meas,idx)

pred_horizon_yaw=30;

yaw0=X_ref_yaw_unbounded(1,idx);
yaw_diff=yaw_meas-yaw0;


yaw_offset=round(yaw_diff/(2*pi))*2*pi;

X_ref_yaw=[X_ref_yaw_unbounded(1,idx:idx+pred_horizon_yaw)+yaw_offset;...
    X_ref_yaw_unbounded(2,idx:idx+pred_horizon_yaw)];

== matlab function FreeFlight Pos Ctrl/Free Flight Reference/create traj/generate_X_ref_z ==
  data: traj_z input double; X_ref_z output double; idx input double
function X_ref_z  = fcn(traj_z,idx)

pred_horizon_z=30;

X_ref_z=traj_z(:,idx:idx+pred_horizon_z);

== matlab function FreeFlight Pos Ctrl/decoupling and rotation/decoupling /Wall Deviation/MATLAB Function ==
  data: u input double; y output double; thres input double
function y = fcn(u,thres)
%#codegen
if u >=thres
    y = 0;
else
    y = u;
end

== matlab function FreeFlight Pos Ctrl/MAIN CONTROL LOOP1/yaw controller MPC FG/MATLAB Function ==
  data: psi_meas input double; psi_prime output double; psi_prev input double
function psi_prime = fcn(psi_meas,psi_prev)
%#codegen

psi_prime = psi_meas;
% 
% if((abs(psi_meas - psi_prev)>= (pi-0.1))&&(psi_prev > 0))
%     psi_prime = pi + abs(pi - abs(psi_meas));
% end
% 
% if((abs(psi_meas - psi_prev)>= (pi-0.1))&&(psi_prev < 0))
%     psi_prime = -pi - abs(pi - abs(psi_meas));
% end


% if((psi_meas>=((45)/180)*pi)&&(psi_meas<=(pi)))
%     psi_prime = (psi_meas - pi) -(180/180)*pi;
% end


end

== matlab function FreeFlight Pos Ctrl/MAIN CONTROL LOOP1/yaw states estimator bias/discrete kalman filter ==
  data: A input double; B input double; state_est output double; C input double; D input double; Q input double; R input double; u input double; y input double; P input double; state input double; P_est output double
function [state_est,P_est]  = fcn(A,B,C,D,Q,R, u, y, P, state)
%#eml

% Kalman filter according to Welch & Bishop, An Introduction to the Kalman
% Filter

n=size(A,1);

% Time update
x_=A*state+B*u;
P_=A*P*A'+Q;
  
% Measurement update
K=P_*C'*(C*P_*C'+R)^-1;
state_est=x_+K*(y-C*x_);
P_est=(eye(n)-K*C)*P_;

== matlab function FreeFlight Pos Ctrl/MAIN CONTROL LOOP1/yaw states estimator bias/MATLAB Function ==
  data: psi_meas input double; psi_prime output double
function psi_prime = fcn(psi_meas)
%#codegen

psi_prime = psi_meas;


if((psi_meas>=((45)/180)*pi)&&(psi_meas<=(pi+0.0175*6.5)))
    psi_prime = (psi_meas - pi) -(180/180)*pi;
end

% if(psi_meas<=pi


end

== matlab function pos controller/MAIN CONTROL LOOP1/yaw states estimator bias/discrete kalman filter ==
  data: A input double; B input double; state_est output double; C input double; D input double; Q input double; R input double; u input double; y input double; P input double; state input double; P_est output double
function [state_est,P_est]  = fcn(A,B,C,D,Q,R, u, y, P, state)
%#eml

% Kalman filter according to Welch & Bishop, An Introduction to the Kalman
% Filter

n=size(A,1);

% Time update
x_=A*state+B*u;
P_=A*P*A'+Q;
  
% Measurement update
K=P_*C'*(C*P_*C'+R)^-1;
state_est=x_+K*(y-C*x_);
P_est=(eye(n)-K*C)*P_;

== matlab function FreeFlight Pos Ctrl/MAIN CONTROL LOOP1/yaw controller MPC FG/MATLAB Function1 ==
  data: psi_meas input double; psi_out output double; x_pos input double; x_w input double; thres_x input double; ref_yaw input double; delta_x output double
function [psi_out,delta_x] = fcn(psi_meas,x_pos,x_w,thres_x,ref_yaw)
%#codegen

psi_out = psi_meas;

if(x_w - x_pos<=thres_x)
    psi_out = ref_yaw;
end

delta_x = x_w - x_pos;

end

== matlab function FreeFlight Pos Ctrl/Subsystem/Wall Point Reference/create traj1/generate_X_ref_x ==
  data: traj_x input double; X_ref_x output double; idx input double
function X_ref_x  = fcn(traj_x,idx)

pred_horizon_x=30;

X_ref_x=traj_x(:,idx:idx+pred_horizon_x);

== matlab function FreeFlight Pos Ctrl/Subsystem/Wall Point Reference/create traj1/generate_X_ref_y ==
  data: traj_y input double; X_ref_y output double; idx input double
function X_ref_y  = fcn(traj_y,idx)

pred_horizon_y=30;

X_ref_y=traj_y(:,idx:idx+pred_horizon_y);

== matlab function FreeFlight Pos Ctrl/Subsystem/Wall Point Reference/create traj1/generate_X_ref_yaw ==
  data: X_ref_yaw_unbounded input double; X_ref_yaw output double; yaw_meas input double; idx input double
function X_ref_yaw  = fcn(X_ref_yaw_unbounded,yaw_meas,idx)

pred_horizon_yaw=30;

yaw0=X_ref_yaw_unbounded(1,idx);
yaw_diff=yaw_meas-yaw0;


yaw_offset=round(yaw_diff/(2*pi))*2*pi;

X_ref_yaw=[X_ref_yaw_unbounded(1,idx:idx+pred_horizon_yaw)+yaw_offset;...
    X_ref_yaw_unbounded(2,idx:idx+pred_horizon_yaw)];

== matlab function FreeFlight Pos Ctrl/Subsystem/Wall Point Reference/create traj1/generate_X_ref_z ==
  data: traj_z input double; X_ref_z output double; idx input double
function X_ref_z  = fcn(traj_z,idx)

pred_horizon_z=30;

X_ref_z=traj_z(:,idx:idx+pred_horizon_z);

== matlab function FreeFlight Pos Ctrl/Subsystem/Wall Point Reference/Next Ref ==
  data: dx input double; y input double; z input double; yref input double; zref input double; thresy input double; thresz input double; threszdown input double; en output double; numSamples input double; counter input double
function en = fcn(dx,y,z,yref,zref,thresy,thresz,threszdown,numSamples,counter)

if abs(y-yref) > thresy
    dy = 1;
else
    dy = 0; % in position
end

% if abs(z-zref) > thresz
%     dz = 1;
% else
%     dz = 0; % in position
% end



if ( (z-zref) > thresz || -(z - zref) > threszdown ) 
    dz = 1;
else
    dz = 0; % in position
end


if dy ~= 0 || dz ~= 0 || dx ~=0
    en = 0; % not yet in position, don't change reference
else
    if counter < numSamples
        en = 1; % in position, both deviations < thres, change ref. point.
    else
        en = 0;
    end
end

== matlab function FreeFlight Pos Ctrl/MAIN CONTROL LOOP1/x controller MPC FG 1/Wall Deviation/MATLAB Function ==
  data: u input double; y output double; thres input double
function y = fcn(u,thres)
%#codegen
if u >=thres
    y = 0;
else
    y = u;
end

== matlab function FreeFlight Pos Ctrl/MAIN CONTROL LOOP1/x controller MPC FG 1/Explicit Ctrl Free Flight1/Subsystem/MATLAB Function ==
  data: state_cur input double; U_x output double; Uprev input double; Mprev input double; nx input double; nu input double; H input double; K input double; Hobj input double; Fobj input double; Gobj input double; F input double; G input double; Nc input double; Qopt input double; Ropt input double; Ml input double; Mr input double; U_y output double; flag_oob output double; M output double
function [U_x,U_y,flag_oob,M] = fcn(state_cur,Uprev,Mprev,nx,nu,H,K,Hobj,Fobj,Gobj,F,G,Nc,Qopt,Ropt,Ml,Mr)
%#codegen

[U,flag_oob,M] = OptimalMPCInputExportC_vP(state_cur,Uprev,Mprev,nx,nu,H,K,Hobj,Fobj,Gobj,F,G,Nc,Qopt,Ropt,Ml,Mr);

U_x = U(1);
U_y = U(2);

end
